simulink model "high"  (R2014a)
settings: Solver=FixedStepDiscrete  StartTime=0.0  StopTime=SimLength  FixedStep=sample_time  RelTol=1e-3
undefined symbols (not defined in the file): SimLength
libraries: simulink x3, dspswit3 x1
settings Model: Creator=Maik  LastModifiedBy=Maik

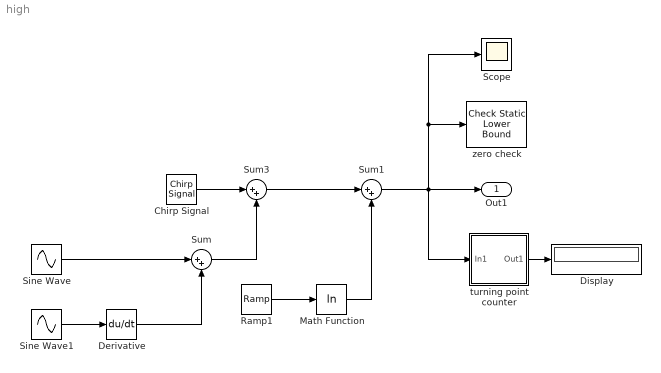
== system high ==
  Chirp Signal : simulink/Sources/Chirp Signal  f1=0.2  T=SimLength  f2=0.7
  Derivative : Derivative
  Display : Display
  Math Function : Math  Operator=log  SaturateOnIntegerOverflow=on
  Ramp1 : simulink/Sources/Ramp  slope=1  start=0  X0=1
  Scope : Scope
      settings: YMin=-1  YMax=1  SaveName=ScopeData5
  Sine Wave : Sin  Amplitude=0.2
  Sine Wave1 : Sin  Amplitude=0.2  Frequency=sqrt(3)
  Sum : Sum  Inputs=|++
  Sum1 : Sum  Inputs=|++
  Sum3 : Sum  Inputs=|++
  turning point counter : Subsystem
  zero check : simulink/Model Verification/Check Static  Lower Bound  Description=0 <= u  min=0  min_included=on  enabled=on  stopWhenAssertionFail=on  export=off  icon=text
  Out1 : Outport
  wires:
  Sine Wave1/1 -> Derivative/1
  Sine Wave/1 -> Sum/1
  Derivative/1 -> Sum/2
  Sum1/1 -> turning point counter/1(In1), Out1/1, Scope/1, zero check/1
  Ramp1/1 -> Math Function/1
  Math Function/1 -> Sum1/2
  Chirp Signal/1 -> Sum3/1
  Sum/1 -> Sum3/2
  Sum3/1 -> Sum1/1
  turning point counter/1(Out1) -> Display/1

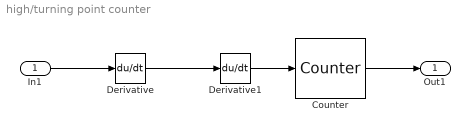
== system high/turning point counter ==
  In1 : Inport
  Counter : dspswit3/Counter  Direction=Up  CountEvent=Either edge  CounterSize=16 bits  MaxCount=255  InitialCount=0  Output=Count  HitValue=0  ResetInput=off  SamplesPerFrame=1  Ts=1  CntDtype=single  HitDtype=Logical
  Derivative : Derivative
  Derivative1 : Derivative
  Out1 : Outport
  wires:
  In1/1 -> Derivative/1
  Derivative/1 -> Derivative1/1
  Derivative1/1 -> Counter/1
  Counter/1 -> Out1/1
